simulink model "Movimiento_TR"  (R2024b)
settings: Solver=ode45  StartTime=0.0  StopTime=10  RelTol=1e-3
model workspace (MAT data in the model file):
  b1 = 1000
  f = 0
  k1 = 16182
  k2 = 19000
  m1 = 290
  m2 = 59
settings Model: Creator=DELL  LastModifiedBy=DELL

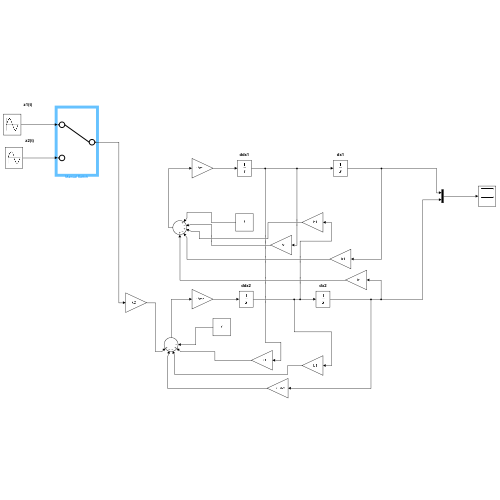
[thumbnail: Simulink's stored preview of the top-level diagram]
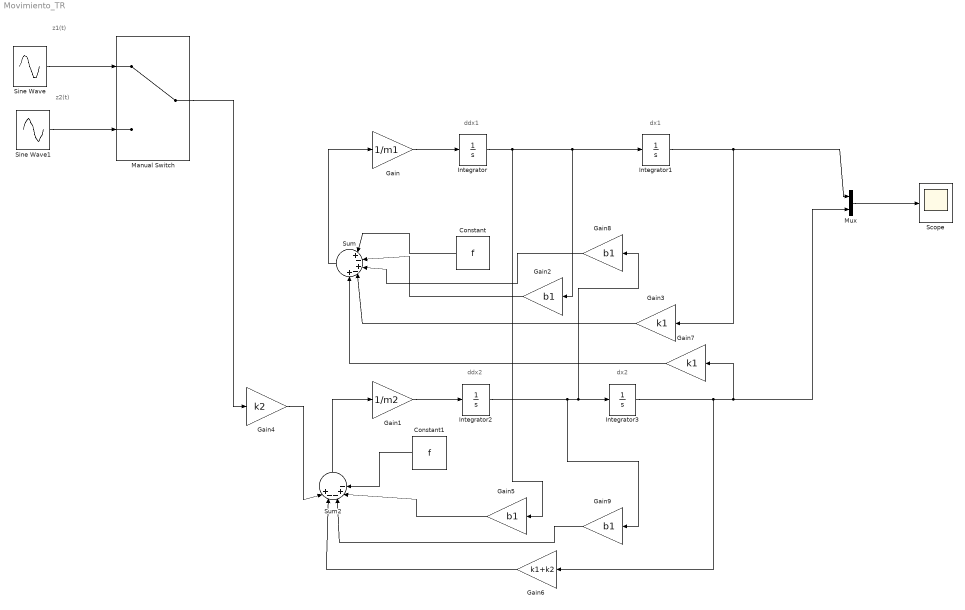
== system Movimiento_TR ==
  note: ddx1
  note: dx1
  note: ddx2
  note: dx2
  note: z1(t)
  note: z2(t)
  Constant : Constant  Value=f
  Constant1 : Constant  Value=f
  Gain : Gain  Gain=1/m1
  Gain1 : Gain  Gain=1/m2
  Gain{2,5,8..9} (4 alike) : Gain  Gain=b1
  Gain3 : Gain  Gain=k1
  Gain4 : Gain  Gain=k2
  Gain6 : Gain  Gain=k1+k2
  Gain7 : Gain  Gain=k1
  Integrator{,1..3} (4 alike) : Integrator
  Manual Switch : ManualSwitch
  Mux : Mux  Inputs=2
  Scope : Scope
  Sine Wave : Sin  Amplitude=0.05  Frequency=0.5*pi  SampleTime=0
  Sine Wave1 : Sin  Amplitude=0.05  Frequency=20*pi  SampleTime=0
  Sum : Sum  Inputs=|+-+-+
  Sum2 : Sum  Inputs=|+--+-
  wires:
  Integrator/1 -> Gain5/1, Gain2/1, Integrator1/1
  Gain/1 -> Integrator/1
  Sum/1 -> Gain/1
  Gain1/1 -> Integrator2/1
  Sum2/1 -> Gain1/1
  Integrator1/1 -> Gain3/1, Mux/1
  Mux/1 -> Scope/1
  Sine Wave/1 -> Manual Switch/1
  Integrator3/1 -> Gain6/1, Gain7/1, Mux/2
  Sine Wave1/1 -> Manual Switch/2
  Manual Switch/1 -> Gain4/1
  Constant/1 -> Sum/1
  Integrator2/1 -> Gain9/1, Gain8/1, Integrator3/1
  Gain4/1 -> Sum2/1
  Gain6/1 -> Sum2/2
  Gain3/1 -> Sum/4
  Constant1/1 -> Sum2/5
  Gain7/1 -> Sum/5
  Gain9/1 -> Sum2/3
  Gain2/1 -> Sum/2
  Gain8/1 -> Sum/3
  Gain5/1 -> Sum2/4
